simulink model "pid_enhanced1"  (Simulink 6.0)
settings: Solver=ode45  StartTime=0.0  StopTime=30  RelTol=1e-3
undefined symbols (not defined in the file): DiscIntNeverNeededParam
settings Model: LastModifiedBy=star

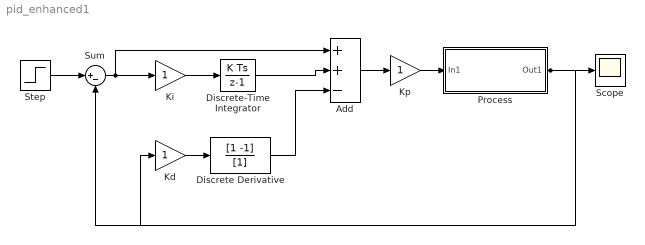
== system pid_enhanced1 ==
  Add : Sum  Inputs=++-  OutScaling=2^-10
  Discrete Derivative : DiscreteFilter  Numerator=[1 -1]  Denominator=[1]
  Discrete-Time Integrator : DiscreteIntegrator  ICPrevOutput=DiscIntNeverNeededParam  ICPrevScaledInput=DiscIntNeverNeededParam
  Kd : Gain
  Ki : Gain
  Kp : Gain
  Process : Subsystem
  Scope : Scope
  Step : Step  Time=0  SampleTime=0
  Sum : Sum  Inputs=|+-
  wires:
  Sum/1 -> Ki/1, Add/1
  Discrete-Time Integrator/1 -> Add/2
  Ki/1 -> Discrete-Time Integrator/1
  Add/1 -> Kp/1
  Kp/1 -> Process/1(In1)
  Process/1(Out1) -> Sum/2, Kd/1, Scope/1
  Kd/1 -> Discrete Derivative/1
  Discrete Derivative/1 -> Add/3
  Step/1 -> Sum/1

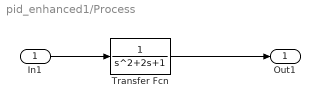
== system pid_enhanced1/Process ==
  In1 : Inport  Port=1  LatchInput=off
  Transfer Fcn : TransferFcn
  Out1 : Outport
  wires:
  In1/1 -> Transfer Fcn/1
  Transfer Fcn/1 -> Out1/1
